simulink model "propeller_modelbased_control_start"  (R2021b)
settings: Solver=VariableStepAuto  StartTime=0.0  StopTime=Inf  RelTol=1e-3
undefined symbols (not defined in the file or in its folder): J, km, L, R, Vmax
settings Model: Creator=cirie  LastModifiedBy=cirie

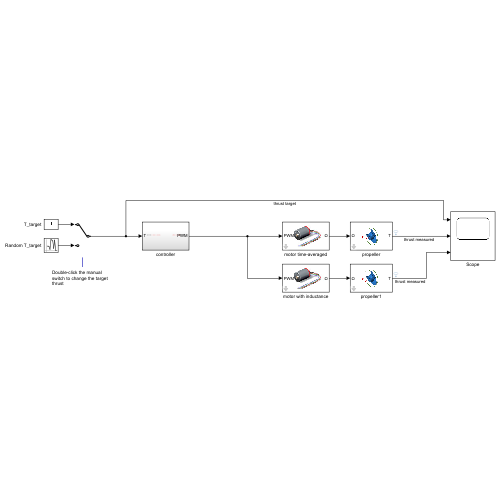
[thumbnail: Simulink's stored preview of the top-level diagram]
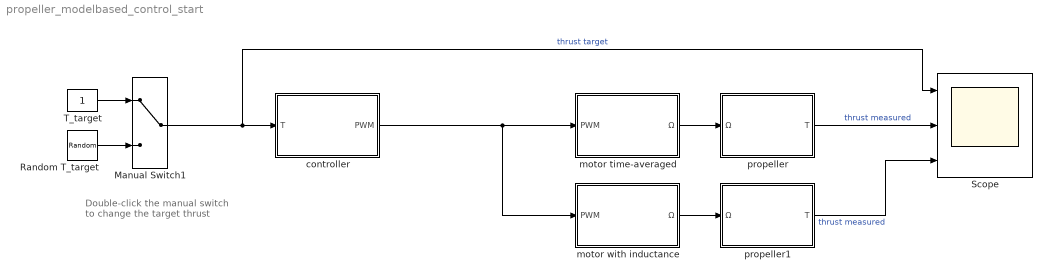
== system propeller_modelbased_control_start ==
  note: Double-click the manual switch to change the target thrust
  Manual Switch1 : ManualSwitch
  Random T_target : RandomNumber  Mean=1  Variance=0.25  SampleTime=1
  Scope : Scope  NumInputPorts=3
  T_target : Constant
  controller : Subsystem
  motor time-averaged : Subsystem  mask(DC Motor){J=1e-4, km=0.1, R=1, Vmax=7.2}
      mask prompts: J "Inertia, J [kgm^2]"; km "Motor constant, km [V*s/rad]"; R "Resistance, R [Ohm]"; Vmax "Maximum Voltage, Vmax [V]"
      mask help:
      | Circuit Dynamics:   PWM*Vmax == I*R + km*Ω
      | Rotor Dynamics:     J*dΩ/dt == km*I
      mask Display: image('$imagefile'); % Use "Edit Image" on toolstrip to change.
  motor with inductance : Subsystem  mask(DC Motor){J=J, km=km, R=R, L=L, Vmax=Vmax}
      mask prompts: J "Inertia, J [kgm^2]"; km "Motor constant, km [V*s/rad]"; R "Resistance, R [Ohm]"; L "Inductance, L [H]"; Vmax "Maximum Voltage, Vmax [V]"
      mask help:
      | Circuit Dynamics:   PWM*Vmax == I*R + km*Ω
      | Rotor Dynamics:     J*dΩ/dt == km*I
      mask Display: image('$imagefile'); % Use "Edit Image" on toolstrip to change.
  propeller : Subsystem  mask(Propeller Model){D=0.1, kt=0.01, rho=1000}
      mask prompts: D "Propeller Diameter [m]"; kt "Thrust Coefficient"; rho "Fluid density [kg/m^3]"
      mask help: Propeller Dynamics: T = kt*rho*omega^2*D^4
      mask Display: image('$imagefile'); % Use "Edit Image" on toolstrip to change.
  propeller1 : Subsystem  mask(Propeller Model){D=0.1, kt=0.01, rho=1000}
      mask prompts: D "Propeller Diameter [m]"; kt "Thrust Coefficient"; rho "Fluid density [kg/m^3]"
      mask help: Propeller Dynamics: T = kt*rho*omega^2*D^4
      mask Display: image('$imagefile'); % Use "Edit Image" on toolstrip to change.
  wires:
  propeller/1(T) -> Scope/2  "thrust measured"
  Manual Switch1/1 -> controller/1(T), Scope/1  "thrust target"
  motor time-averaged/1(Ω) -> propeller/1(Ω)
  controller/1(PWM) -> motor with inductance/1(PWM), motor time-averaged/1(PWM)
  Random T_target/1 -> Manual Switch1/2
  T_target/1 -> Manual Switch1/1
  motor with inductance/1(Ω) -> propeller1/1(Ω)
  propeller1/1(T) -> Scope/3  "thrust measured"

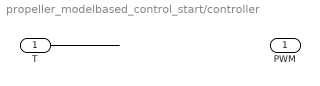
== system propeller_modelbased_control_start/controller ==
  T : Inport
  PWM : Outport
  wires:
  T/1 -> ?
  ? -> PWM/1

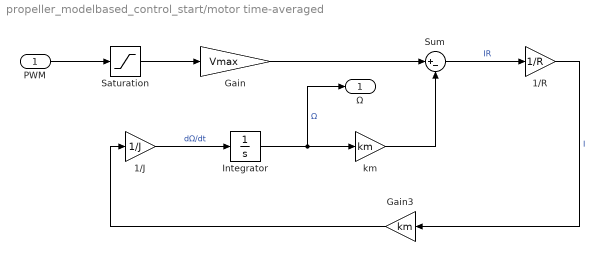
== system propeller_modelbased_control_start/motor time-averaged ==
  PWM : Inport
  1/J : Gain  Gain=1/J
  1/R : Gain  Gain=1/R
  Gain : Gain  Gain=Vmax
  Gain3 : Gain  Gain=km
  Integrator : Integrator
  Saturation : Saturate  UpperLimit=1  LowerLimit=-1
  Sum : Sum  Inputs=|+-
  km : Gain  Gain=km
  Ω : Outport
  wires:
  1/J/1 -> Integrator/1  "dΩ/dt"
  Sum/1 -> 1/R/1  "IR"
  Integrator/1 -> Ω/1, km/1  "Ω"
  Gain3/1 -> 1/J/1
  km/1 -> Sum/2
  1/R/1 -> Gain3/1  "I"
  PWM/1 -> Saturation/1
  Gain/1 -> Sum/1
  Saturation/1 -> Gain/1

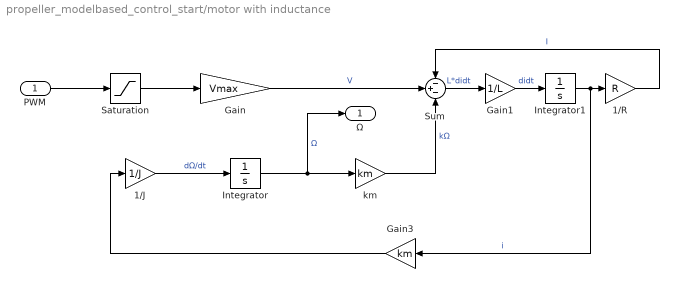
== system propeller_modelbased_control_start/motor with inductance ==
  PWM : Inport
  1/J : Gain  Gain=1/J
  1/R : Gain  Gain=R
  Gain : Gain  Gain=Vmax
  Gain1 : Gain  Gain=1/L
  Gain3 : Gain  Gain=km
  Integrator : Integrator
  Integrator1 : Integrator
  Saturation : Saturate  UpperLimit=1  LowerLimit=-1
  Sum : Sum  Inputs=-+-
  km : Gain  Gain=km
  Ω : Outport
  wires:
  1/J/1 -> Integrator/1  "dΩ/dt"
  Integrator1/1 -> Gain3/1, 1/R/1  "i"
  Integrator/1 -> Ω/1, km/1  "Ω"
  Gain3/1 -> 1/J/1
  km/1 -> Sum/3  "kΩ"
  1/R/1 -> Sum/1  "I"
  PWM/1 -> Saturation/1
  Gain/1 -> Sum/2  "V"
  Saturation/1 -> Gain/1
  Sum/1 -> Gain1/1  "L*didt"
  Gain1/1 -> Integrator1/1  "didt"

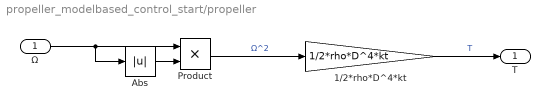
== system propeller_modelbased_control_start/propeller ==
  Ω : Inport
  1/2*rho*D^4*kt : Gain  Gain=1/2*rho*D^4*kt
  Abs : Abs
  Product : Product
  T : Outport
  wires:
  1/2*rho*D^4*kt/1 -> T/1  "T"
  Product/1 -> 1/2*rho*D^4*kt/1  "Ω^2"
  Ω/1 -> Abs/1, Product/1
  Abs/1 -> Product/2

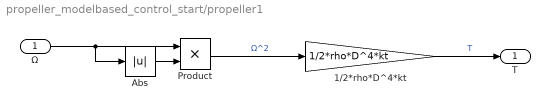
== system propeller_modelbased_control_start/propeller1 ==
  Ω : Inport
  1/2*rho*D^4*kt : Gain  Gain=1/2*rho*D^4*kt
  Abs : Abs
  Product : Product
  T : Outport
  wires:
  Abs/1 -> Product/2
  Ω/1 -> Product/1, Abs/1
  Product/1 -> 1/2*rho*D^4*kt/1  "Ω^2"
  1/2*rho*D^4*kt/1 -> T/1  "T"
